simulink model "uz_interlockDeadtime2L"  (R2023a)
settings: Solver=FixedStepDiscrete  StartTime=0.0  StopTime=0.003  RelTol=1e-3
undefined symbols (not defined in the file or in its folder): f_FPGA_clk, T_FPGA_clk
libraries: simulink x3, hdlsllib x3
(part 1 of 2)
settings Model: DataTypeOverride=Off  Creator=ts  LastModifiedBy=ts
settings SolverCC: AlgebraicLoopSolver=TrustRegion
settings DataIOCC: LimitDataPoints=on  SaveOutput=off  SaveTime=off
settings OptimizationCC: BlockReduction=off  ConditionallyExecuteInputs=off  DefaultParameterBehavior=Inlined  LifeSpan=inf
settings DebuggingCC: AlgebraicLoopMsg=error  SingleTaskRateTransMsg=error  UnconnectedInputMsg=warning  UnconnectedOutputMsg=warning  UnconnectedLineMsg=warning  AllowSymbolicDim=off  StrictBusMsg=ErrorOnBusTreatedAsVector  SFUnexpectedBacktrackingDiag=warning  SFNoUnconditionalDefaultTransitionDiag=warning  SFExecutionAtInitializationDiag=none  ArithmeticOperatorsInVariantConditions=warning
settings HardwareCC: ProdBitPerPointer=32  ProdBitPerSizeT=32  ProdBitPerPtrDiffT=32  ProdLargestAtomicFloat=None  ProdIntDivRoundTo=Undefined  ProdEndianess=Unspecified  ProdWordSize=32  ProdHWDeviceType=ASIC/FPGA->ASIC/FPGA  ProdEqTarget=off
settings ModelReferenceCC: EnableRefExpFcnMdlSchedulingChecks=on
settings SFSimCC: SimUseLocalCustomCode=off  CustomCodeUndefinedFunction=UseInterfaceOnly
settings RTWCC: RTWUseLocalCustomCode=off  DLArmComputeVersion=19.05
settings CodeAppCC: StateflowObjectComments=on
settings GRTTargetCC: TargetLangStandard=C89/C90 (ANSI)
settings ConfigComp: CovScope=ReferencedModels  CovMetricSettings=dw  CovSaveCumulativeToWorkspaceVar=on  CovSaveSingleToWorkspaceVar=on  CovExternalEMLEnable=off  CovSFcnEnable=off

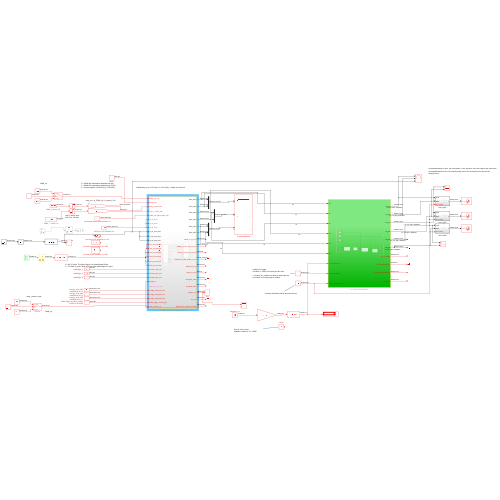
[thumbnail: Simulink's stored preview of the top-level diagram]
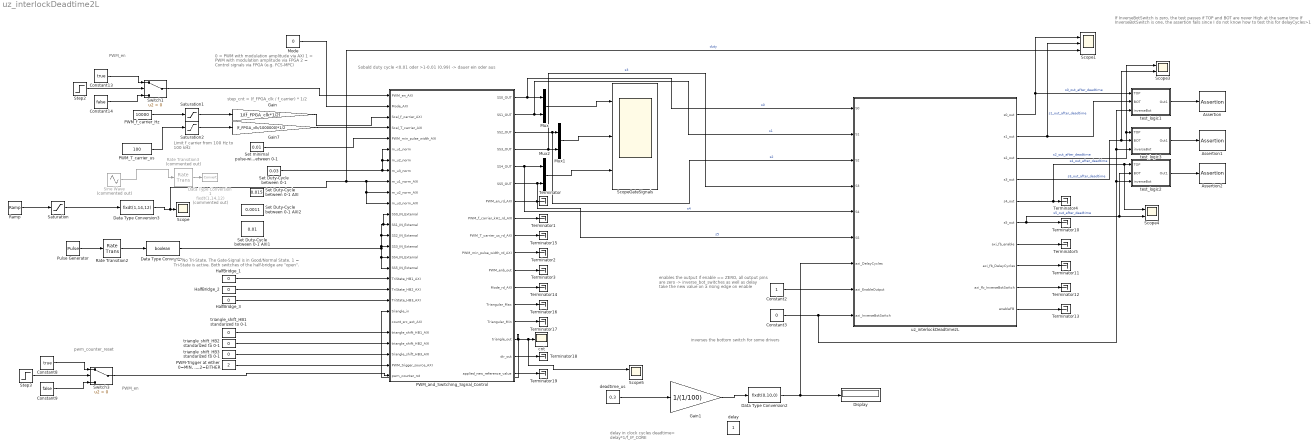
== system uz_interlockDeadtime2L ==
  note: Sobald duty cycle <0.01 oder >1-0.01 (0.99) -> dauer ein oder aus
  note: If InverseBotSwitch is zero, the test passes if TOP and BOT are never High at the same time
      | If InverseBotSwitch is one, the assertion fails since I do not know how to test this for delayCycles>1
  note: enables the output
      | if enable == ZERO, all output pins are zero
      |
      | -> inverse_bot_switches as well as delay take the
      | new value on a rising edge on enable
  note: inverses the bottom switch for some drivers
  note: delay in clock cycles
      | deadtime= delay*1/f_IP_CORE
  note: 0 = No Tri-State. The Gate-Signal is in Good/Normal State.
      | 1 = Tri-State is active. Both switches of the half-bridge are "open".
  note: 0 = PWM with modulation amplitude via AXI
      | 1 = PWM with modulation amplitude via FPGA
      | 2 = Control signals via FPGA (e.g. FCS-MPC)
  note: PWM_en
  note: Limit f_carrier from
      | 100 Hz to 100 kHz
  note: PWM_en
  note: step_cnt = (f_FPGA_clk / f_carrier) * 1/2
  note: pwm_counter_reset
  Assertion : Assertion
  Assertion1 : Assertion
  Assertion2 : Assertion
  Constant13 : Constant  Value=true  SampleTime=T_FPGA_clk
  Constant14 : Constant  Value=false  SampleTime=T_FPGA_clk
  Constant2 : Constant  OutDataTypeStr=boolean  SampleTime=1/100e6
  Constant3 : Constant  Value=0  OutDataTypeStr=boolean  SampleTime=1/100e6
  Constant8 : Constant  Value=true  SampleTime=T_FPGA_clk
  Constant9 : Constant  Value=false  SampleTime=T_FPGA_clk
  Data Type Conversion : DataTypeConversion  OutDataTypeStr=boolean  SaturateOnIntegerOverflow=off  RndMeth=Floor
  Data Type Conversion1 : DataTypeConversion  Commented=on  OutDataTypeStr=fixdt(1,14,12)  SaturateOnIntegerOverflow=off  RndMeth=Floor
  Data Type Conversion2 : DataTypeConversion  OutDataTypeStr=fixdt(0,10,0)  SaturateOnIntegerOverflow=off  RndMeth=Floor
  Data Type Conversion3 : DataTypeConversion  OutDataTypeStr=fixdt(1,14,12)  SaturateOnIntegerOverflow=off  RndMeth=Floor
  Display : Display
  Gain : Gain  Gain=1/(f_FPGA_clk*1/2)  OutDataTypeStr=fixdt(0,25,26)
  Gain1 : Gain  Gain=1/(1/100)
  Gain7 : Gain  Gain=(f_FPGA_clk/1000000)*1/2  OutDataTypeStr=fixdt(0,25,0)
  HalfBridge_1 : Constant  Value=0  OutDataTypeStr=fixdt(0,2,0)  SampleTime=T_FPGA_clk
  HalfBridge_2 : Constant  Value=0  OutDataTypeStr=fixdt(0,2,0)  SampleTime=T_FPGA_clk
  HalfBridge_3 : Constant  Value=0  OutDataTypeStr=fixdt(0,2,0)  SampleTime=T_FPGA_clk
  Mode : Constant  Value=0  OutDataTypeStr=fixdt(0,2,0)  SampleTime=T_FPGA_clk
  Mux : Mux  Inputs=2
  Mux1 : Mux  Inputs=2
  Mux2 : Mux  Inputs=2
  "PWM-Trigger at either 0=MIN, 1=MAX,2=EITHER" : Constant  Value=2  OutDataTypeStr=uint32  SampleTime=T_FPGA_clk
  PWM_T_carrier_us : Constant  Value=100  OutDataTypeStr=uint32  SampleTime=T_FPGA_clk
  PWM_and_Switching_Signal_Control : Subsystem  TreatAsAtomicUnit=on
  PWM_f_carrier_Hz : Constant  Value=10000  OutDataTypeStr=uint32  SampleTime=T_FPGA_clk
  Pulse Generator : DiscretePulseGenerator  PulseType=Time based  Period=0.01  PulseWidth=5
  Ramp : simulink/Sources/Ramp  slope=0.0000001/T_FPGA_clk  start=T_FPGA_clk  InitialOutput=0.97
  Rate Transition2 : RateTransition  OutPortSampleTime=T_FPGA_clk
  Rate Transition3 : RateTransition  Commented=on  OutPortSampleTime=T_FPGA_clk
  Saturation : Saturate  UpperLimit=1  LowerLimit=0
  Saturation1 : Saturate  UpperLimit=100000  LowerLimit=100
  Saturation2 : Saturate  UpperLimit=10000  LowerLimit=10
  Scope : Scope
  Scope1 : Scope  NumInputPorts=3
  Scope3 : Scope  NumInputPorts=2
  Scope4 : Scope  NumInputPorts=2
  Scope5 : Scope  NumInputPorts=2
  ScopeGateSignals : Scope  NumInputPorts=3
  Set Duty-Cycle between 0-1 : Constant  Value=0.03  OutDataTypeStr=fixdt(1,14,12)  SampleTime=T_FPGA_clk
  Set Duty-Cycle between 0-1 AXI : Constant  Value=0.015  OutDataTypeStr=fixdt(1,14,12)  SampleTime=T_FPGA_clk
  Set Duty-Cycle between 0-1 AXI1 : Constant  Value=0.01  OutDataTypeStr=fixdt(1,14,12)  SampleTime=T_FPGA_clk
  Set Duty-Cycle between 0-1 AXI2 : Constant  Value=0.0011  OutDataTypeStr=fixdt(1,14,12)  SampleTime=T_FPGA_clk
  Set minimal pulse-width between 0-1 : Constant  Value=0.01  OutDataTypeStr=fixdt(1,18,16)  SampleTime=T_FPGA_clk
  Sine Wave : Sin  Commented=on  Frequency=500  SampleTime=0
  Step2 : Step  Time=0.002  Before=1  SampleTime=T_FPGA_clk
  Step3 : Step  Time=0.00025  After=0  SampleTime=T_FPGA_clk
  Switch1 : Switch  Criteria=u2 > Threshold  SaturateOnIntegerOverflow=off  InputSameDT=off
  Switch3 : Switch  Criteria=u2 > Threshold  SaturateOnIntegerOverflow=off  InputSameDT=off
  Terminator{,1..5,10..19} (16 alike) : Terminator
  cnt : Scope
  deadtime_us : Constant  Value=0.3  OutDataTypeStr=double  SampleTime=1/100e6
  delay : Constant  OutDataTypeStr=fixdt(0,10,0)  SampleTime=1/100e6
  test_logic1 : Subsystem
  test_logic2 : Subsystem
  test_logic3 : Subsystem
  triangle_shift_HB1 standarized to 0-1 : Constant  Value=0  OutDataTypeStr=fixdt(0,18,17)  SampleTime=T_FPGA_clk
  triangle_shift_HB2 standarized to 0-1 : Constant  Value=0  OutDataTypeStr=fixdt(0,18,17)  SampleTime=T_FPGA_clk
  triangle_shift_HB3 standarized to 0-1 : Constant  Value=0  OutDataTypeStr=fixdt(0,18,17)  SampleTime=T_FPGA_clk
  uz_interlockDeadtime2L : Subsystem  TreatAsAtomicUnit=on
  wires:
  Constant2/1 -> uz_interlockDeadtime2L/8(axi_EnableOutput)
  uz_interlockDeadtime2L/1(s0_out) -> Scope1/1, test_logic1/1(TOP)  "s0_out_after_deadtime"
  uz_interlockDeadtime2L/2(s1_out) -> Scope1/2, test_logic1/2(BOT)  "s1_out_after_deadtime"
  uz_interlockDeadtime2L/3(s2_out) -> Scope3/1, test_logic3/1(TOP)  "s2_out_after_deadtime"
  uz_interlockDeadtime2L/4(s3_out) -> Scope3/2, test_logic3/2(BOT)  "s3_out_after_deadtime"
  uz_interlockDeadtime2L/5(s4_out) -> Scope4/1, test_logic2/1(TOP), Terminator4/1  "s4_out_after_deadtime"
  Constant3/1 -> uz_interlockDeadtime2L/9(axi_InverseBotSwitch), test_logic2/3(inverseBot), test_logic3/3(inverseBot), test_logic1/3(inverseBot)
  uz_interlockDeadtime2L/6(s5_out) -> test_logic2/2(BOT), Scope4/2, Terminator10/1  "s5_out_after_deadtime"
  uz_interlockDeadtime2L/7(axi_fb_enable) -> Terminator5/1
  uz_interlockDeadtime2L/8(axi_fb_DelayCycles) -> Terminator11/1
  uz_interlockDeadtime2L/9(axi_fb_InverseBotSwitch) -> Terminator12/1
  uz_interlockDeadtime2L/10(enableFB) -> Terminator13/1
  test_logic3/1(Out1) -> Assertion1/1
  test_logic2/1(Out1) -> Assertion2/1
  test_logic1/1(Out1) -> Assertion/1
  Data Type Conversion2/1 -> Display/1, uz_interlockDeadtime2L/7(axi_DelayCycles)
  PWM_and_Switching_Signal_Control/13(Triangular_Max) -> Terminator16/1
  triangle_shift_HB3 standarized to 0-1/1 -> PWM_and_Switching_Signal_Control/25(triangle_shift_HB3_AXI)
  PWM_and_Switching_Signal_Control/8(PWM_f_carrier_kHz_rd_AXI) -> Terminator1/1
  triangle_shift_HB1 standarized to 0-1/1 -> PWM_and_Switching_Signal_Control/23(triangle_shift_HB1_AXI)
  PWM_and_Switching_Signal_Control/7(PWM_en_rd_AXI) -> Terminator/1
  PWM_and_Switching_Signal_Control/15(triangle_out) -> PWM_and_Switching_Signal_Control/21(triangle_in), Scope5/1, cnt/1
  PWM_and_Switching_Signal_Control/2(SS1_OUT) -> uz_interlockDeadtime2L/2(S1), Mux/2  "s1"
  Constant9/1 -> Switch3/3
  Constant14/1 -> Switch1/3
  "PWM-Trigger at either 0=MIN, 1=MAX,2=EITHER"/1 -> PWM_and_Switching_Signal_Control/26(PWM_trigger_source_AXI)
  Switch1/1 -> PWM_and_Switching_Signal_Control/1(PWM_en_AXI)
  Set Duty-Cycle between 0-1/1 -> PWM_and_Switching_Signal_Control/6(m_u1_norm), PWM_and_Switching_Signal_Control/7(m_u2_norm), PWM_and_Switching_Signal_Control/8(m_u3_norm)
  Mux/1 -> ScopeGateSignals/1
  Data Type Conversion/1 -> PWM_and_Switching_Signal_Control/13(SS1_IN_External), PWM_and_Switching_Signal_Control/12(SS0_IN_External), PWM_and_Switching_Signal_Control/14(SS2_IN_External), PWM_and_Switching_Signal_Control/15(SS3_IN_External), PWM_and_Switching_Signal_Control/17(SS5_IN_External), PWM_and_Switching_Signal_Control/16(SS4_IN_External)
  Mode/1 -> PWM_and_Switching_Signal_Control/2(Mode_AXI)
  Gain/1 -> PWM_and_Switching_Signal_Control/3(Scal_f_carrier_AXI)
  Pulse Generator/1 -> Rate Transition2/1
  Constant8/1 -> Switch3/1
  PWM_and_Switching_Signal_Control/14(Triangular_Min) -> Terminator17/1
  HalfBridge_3/1 -> PWM_and_Switching_Signal_Control/20(TriState_HB3_AXI)
  Mux2/1 -> ScopeGateSignals/3
  PWM_T_carrier_us/1 -> Saturation2/1
  Saturation2/1 -> Gain7/1
  PWM_and_Switching_Signal_Control/11(PWM_enb_out) -> Terminator3/1
  PWM_and_Switching_Signal_Control/9(PWM_T_carrier_us_rd_AXI) -> Terminator15/1
  Rate Transition3/1 -> Data Type Conversion1/1
  PWM_and_Switching_Signal_Control/12(Mode_rd_AXI) -> Terminator14/1
  PWM_and_Switching_Signal_Control/16(dir_out) -> Terminator18/1
  Rate Transition2/1 -> Data Type Conversion/1
  HalfBridge_1/1 -> PWM_and_Switching_Signal_Control/18(TriState_HB1_AXI)
  PWM_and_Switching_Signal_Control/17(applied_new_reference_value) -> Terminator19/1
  PWM_and_Switching_Signal_Control/4(SS3_OUT) -> uz_interlockDeadtime2L/4(S3), Mux1/2  "s3"
  Mux1/1 -> ScopeGateSignals/2
  PWM_and_Switching_Signal_Control/6(SS5_OUT) -> uz_interlockDeadtime2L/6(S5), Mux2/2  "s5"
  PWM_and_Switching_Signal_Control/10(PWM_min_pulse_width_rd_AXI) -> Terminator2/1
  HalfBridge_2/1 -> PWM_and_Switching_Signal_Control/19(TriState_HB2_AXI)
  Constant13/1 -> Switch1/1
  PWM_and_Switching_Signal_Control/5(SS4_OUT) -> uz_interlockDeadtime2L/5(S4), Mux2/1  "s4"
  Gain7/1 -> PWM_and_Switching_Signal_Control/4(Scal_T_carrier_AXI)
  Step3/1 -> Switch3/2
  Sine Wave/1 -> Rate Transition3/1
  Switch3/1 -> PWM_and_Switching_Signal_Control/27(pwm_counter_rst)
  PWM_and_Switching_Signal_Control/1(SS0_OUT) -> uz_interlockDeadtime2L/1(S0), Mux/1  "s0"
  Data Type Conversion3/1 -> Scope1/3, PWM_and_Switching_Signal_Control/11(m_u3_norm_AXI), PWM_and_Switching_Signal_Control/10(m_u2_norm_AXI), PWM_and_Switching_Signal_Control/9(m_u1_norm_AXI), Scope/1  "duty"
  PWM_and_Switching_Signal_Control/3(SS2_OUT) -> uz_interlockDeadtime2L/3(S2), Mux1/1  "s2"
  triangle_shift_HB2 standarized to 0-1/1 -> PWM_and_Switching_Signal_Control/24(triangle_shift_HB2_AXI)
  Saturation1/1 -> Gain/1
  Step2/1 -> Switch1/2
  PWM_f_carrier_Hz/1 -> Saturation1/1
  Set minimal pulse-width between 0-1/1 -> PWM_and_Switching_Signal_Control/5(PWM_min_pulse_width_AXI)
  deadtime_us/1 -> Gain1/1
  Gain1/1 -> Data Type Conversion2/1
  Ramp/1 -> Saturation/1
  Saturation/1 -> Data Type Conversion3/1

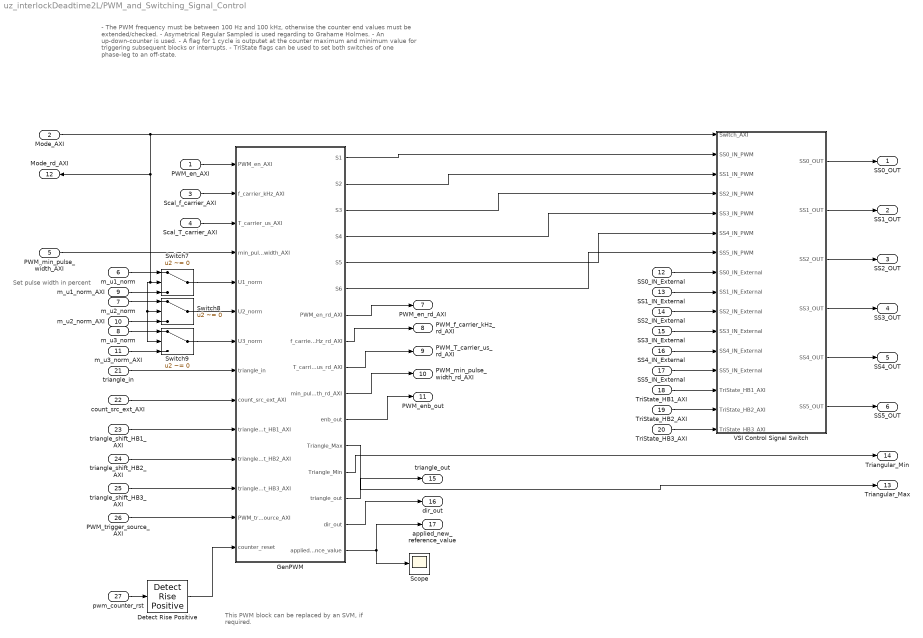
== system uz_interlockDeadtime2L/PWM_and_Switching_Signal_Control ==
  note: This PWM block can be replaced by an SVM,
      | if required.
  note: - The PWM frequency must be between 100 Hz and 100 kHz, otherwise the counter end values must be extended/checked.
      | - Asymetrical Regular Sampled is used regarding to Grahame Holmes.
      | - An up-down-counter is used.
      | - A flag for 1 cycle is outputet at the counter maximum and minimum value for triggering subsequent blocks or interrupts.
      | - TriState flags can be used to set both switches of one phase-leg to an off-state.
  note: Set pulse width in percent
  PWM_en_AXI : Inport
  Mode_AXI : Inport  Port=2
  Scal_f_carrier_AXI : Inport  Port=3
  Scal_T_carrier_AXI : Inport  Port=4
  PWM_min_pulse_width_AXI : Inport  Port=5
  m_u1_norm : Inport  Port=6
  m_u2_norm : Inport  Port=7
  m_u3_norm : Inport  Port=8
  m_u1_norm_AXI : Inport  Port=9
  m_u2_norm_AXI : Inport  Port=10
  m_u3_norm_AXI : Inport  Port=11
  SS0_IN_External : Inport  Port=12
  SS1_IN_External : Inport  Port=13
  SS2_IN_External : Inport  Port=14
  SS3_IN_External : Inport  Port=15
  SS4_IN_External : Inport  Port=16
  SS5_IN_External : Inport  Port=17
  TriState_HB1_AXI : Inport  Port=18
  TriState_HB2_AXI : Inport  Port=19
  TriState_HB3_AXI : Inport  Port=20
  triangle_in : Inport  Port=21
  count_src_ext_AXI : Inport  Port=22
  triangle_shift_HB1_AXI : Inport  Port=23
  triangle_shift_HB2_AXI : Inport  Port=24
  triangle_shift_HB3_AXI : Inport  Port=25
  PWM_trigger_source_AXI : Inport  Port=26
  pwm_counter_rst : Inport  Port=27
  Detect Rise Positive : simulink/Logic and Bit Operations/Detect Rise Positive  vinit=0  OutDataTypeStr=boolean
  GenPWM : Subsystem  TreatAsAtomicUnit=on
  Scope : Scope
  Switch7 : Switch  Criteria=u2 ~= 0  SaturateOnIntegerOverflow=off  InputSameDT=off
  Switch8 : Switch  Criteria=u2 ~= 0  SaturateOnIntegerOverflow=off  InputSameDT=off
  Switch9 : Switch  Criteria=u2 ~= 0  SaturateOnIntegerOverflow=off  InputSameDT=off
  VSI Control Signal Switch : Subsystem
  SS0_OUT : Outport  VectorParamsAs1DForOutWhenUnconnected=off
  SS1_OUT : Outport  Port=2  VectorParamsAs1DForOutWhenUnconnected=off
  SS2_OUT : Outport  Port=3  VectorParamsAs1DForOutWhenUnconnected=off
  SS3_OUT : Outport  Port=4  VectorParamsAs1DForOutWhenUnconnected=off
  SS4_OUT : Outport  Port=5  VectorParamsAs1DForOutWhenUnconnected=off
  SS5_OUT : Outport  Port=6  VectorParamsAs1DForOutWhenUnconnected=off
  PWM_en_rd_AXI : Outport  Port=7  VectorParamsAs1DForOutWhenUnconnected=off
  PWM_f_carrier_kHz_rd_AXI : Outport  Port=8  VectorParamsAs1DForOutWhenUnconnected=off
  PWM_T_carrier_us_rd_AXI : Outport  Port=9  VectorParamsAs1DForOutWhenUnconnected=off
  PWM_min_pulse_width_rd_AXI : Outport  Port=10  VectorParamsAs1DForOutWhenUnconnected=off
  PWM_enb_out : Outport  Port=11  VectorParamsAs1DForOutWhenUnconnected=off
  Mode_rd_AXI : Outport  Port=12  VectorParamsAs1DForOutWhenUnconnected=off
  Triangular_Max : Outport  Port=13  VectorParamsAs1DForOutWhenUnconnected=off
  Triangular_Min : Outport  Port=14  VectorParamsAs1DForOutWhenUnconnected=off
  triangle_out : Outport  Port=15  VectorParamsAs1DForOutWhenUnconnected=off
  dir_out : Outport  Port=16  VectorParamsAs1DForOutWhenUnconnected=off
  applied_new_reference_value : Outport  Port=17  VectorParamsAs1DForOutWhenUnconnected=off
  wires:
  VSI Control Signal Switch/1(SS0_OUT) -> SS0_OUT/1
  Mode_AXI/1 -> Mode_rd_AXI/1, Switch9/2, Switch8/2, Switch7/2, VSI Control Signal Switch/1(Switch_AXI)
  GenPWM/4(S4) -> VSI Control Signal Switch/5(SS3_IN_PWM)
  Scal_f_carrier_AXI/1 -> GenPWM/2(f_carrier_kHz_AXI)
  GenPWM/2(S2) -> VSI Control Signal Switch/3(SS1_IN_PWM)
  SS1_IN_External/1 -> VSI Control Signal Switch/9(SS1_IN_External)
  GenPWM/3(S3) -> VSI Control Signal Switch/4(SS2_IN_PWM)
  GenPWM/5(S5) -> VSI Control Signal Switch/6(SS4_IN_PWM)
  GenPWM/6(S6) -> VSI Control Signal Switch/7(SS5_IN_PWM)
  VSI Control Signal Switch/6(SS5_OUT) -> SS5_OUT/1
  GenPWM/1(S1) -> VSI Control Signal Switch/2(SS0_IN_PWM)
  GenPWM/11(enb_out) -> PWM_enb_out/1
  VSI Control Signal Switch/3(SS2_OUT) -> SS2_OUT/1
  SS3_IN_External/1 -> VSI Control Signal Switch/11(SS3_IN_External)
  SS0_IN_External/1 -> VSI Control Signal Switch/8(SS0_IN_External)
  VSI Control Signal Switch/2(SS1_OUT) -> SS1_OUT/1
  SS4_IN_External/1 -> VSI Control Signal Switch/12(SS4_IN_External)
  PWM_en_AXI/1 -> GenPWM/1(PWM_en_AXI)
  SS5_IN_External/1 -> VSI Control Signal Switch/13(SS5_IN_External)
  VSI Control Signal Switch/5(SS4_OUT) -> SS4_OUT/1
  PWM_min_pulse_width_AXI/1 -> GenPWM/4(min_pulse_width_AXI)
  SS2_IN_External/1 -> VSI Control Signal Switch/10(SS2_IN_External)
  VSI Control Signal Switch/4(SS3_OUT) -> SS3_OUT/1
  Switch9/1 -> GenPWM/7(U3_norm)
  m_u1_norm_AXI/1 -> Switch7/3
  m_u1_norm/1 -> Switch7/1
  m_u2_norm/1 -> Switch8/1
  m_u2_norm_AXI/1 -> Switch8/3
  m_u3_norm/1 -> Switch9/1
  m_u3_norm_AXI/1 -> Switch9/3
  GenPWM/7(PWM_en_rd_AXI) -> PWM_en_rd_AXI/1
  GenPWM/8(f_carrier_kHz_rd_AXI) -> PWM_f_carrier_kHz_rd_AXI/1
  GenPWM/10(min_pulse_width_rd_AXI) -> PWM_min_pulse_width_rd_AXI/1
  GenPWM/9(T_carrier_us_rd_AXI) -> PWM_T_carrier_us_rd_AXI/1
  Switch8/1 -> GenPWM/6(U2_norm)
  Switch7/1 -> GenPWM/5(U1_norm)
  Scal_T_carrier_AXI/1 -> GenPWM/3(T_carrier_us_AXI)
  GenPWM/12(Triangle_Max) -> Triangular_Max/1
  TriState_HB1_AXI/1 -> VSI Control Signal Switch/14(TriState_HB1_AXI)
  TriState_HB2_AXI/1 -> VSI Control Signal Switch/15(TriState_HB2_AXI)
  TriState_HB3_AXI/1 -> VSI Control Signal Switch/16(TriState_HB3_AXI)
  GenPWM/13(Triangle_Min) -> Triangular_Min/1
  triangle_in/1 -> GenPWM/8(triangle_in)
  GenPWM/14(triangle_out) -> triangle_out/1
  GenPWM/15(dir_out) -> dir_out/1
  count_src_ext_AXI/1 -> GenPWM/9(count_src_ext_AXI)
  triangle_shift_HB1_AXI/1 -> GenPWM/10(triangle_shift_HB1_AXI)
  triangle_shift_HB3_AXI/1 -> GenPWM/12(triangle_shift_HB3_AXI)
  triangle_shift_HB2_AXI/1 -> GenPWM/11(triangle_shift_HB2_AXI)
  PWM_trigger_source_AXI/1 -> GenPWM/13(PWM_trigger_source_AXI)
  GenPWM/16(applied_new_reference_value) -> Scope/1, applied_new_reference_value/1
  Detect Rise Positive/1 -> GenPWM/14(counter_reset)
  pwm_counter_rst/1 -> Detect Rise Positive/1

== system uz_interlockDeadtime2L/test_logic1 ==
  TOP : Inport
  BOT : Inport  Port=2
  inverseBot : Inport  Port=3
  AND : Logic  IconShape=distinctive  AllPortsSameDT=off  OutDataTypeStr=boolean
  Constant : Constant
  NOT : Logic  Operator=NOT  IconShape=distinctive  AllPortsSameDT=off  OutDataTypeStr=boolean
  Switch : Switch  Criteria=u2 ~= 0  SaturateOnIntegerOverflow=off  InputSameDT=off
  Out1 : Outport
  wires:
  Constant/1 -> Switch/1
  Switch/1 -> Out1/1
  AND/1 -> NOT/1
  inverseBot/1 -> Switch/2
  NOT/1 -> Switch/3
  TOP/1 -> AND/1
  BOT/1 -> AND/2

== system uz_interlockDeadtime2L/test_logic2 ==
  TOP : Inport
  BOT : Inport  Port=2
  inverseBot : Inport  Port=3
  AND : Logic  IconShape=distinctive  AllPortsSameDT=off  OutDataTypeStr=boolean
  Constant : Constant
  NOT : Logic  Operator=NOT  IconShape=distinctive  AllPortsSameDT=off  OutDataTypeStr=boolean
  Switch : Switch  Criteria=u2 ~= 0  SaturateOnIntegerOverflow=off  InputSameDT=off
  Out1 : Outport
  wires:
  BOT/1 -> AND/2
  TOP/1 -> AND/1
  NOT/1 -> Switch/3
  inverseBot/1 -> Switch/2
  AND/1 -> NOT/1
  Switch/1 -> Out1/1
  Constant/1 -> Switch/1

== system uz_interlockDeadtime2L/test_logic3 ==
  TOP : Inport
  BOT : Inport  Port=2
  inverseBot : Inport  Port=3
  AND : Logic  IconShape=distinctive  AllPortsSameDT=off  OutDataTypeStr=boolean
  Constant : Constant
  NOT : Logic  Operator=NOT  IconShape=distinctive  AllPortsSameDT=off  OutDataTypeStr=boolean
  Switch : Switch  Criteria=u2 ~= 0  SaturateOnIntegerOverflow=off  InputSameDT=off
  Out1 : Outport
  wires:
  Constant/1 -> Switch/1
  Switch/1 -> Out1/1
  AND/1 -> NOT/1
  inverseBot/1 -> Switch/2
  NOT/1 -> Switch/3
  TOP/1 -> AND/1
  BOT/1 -> AND/2

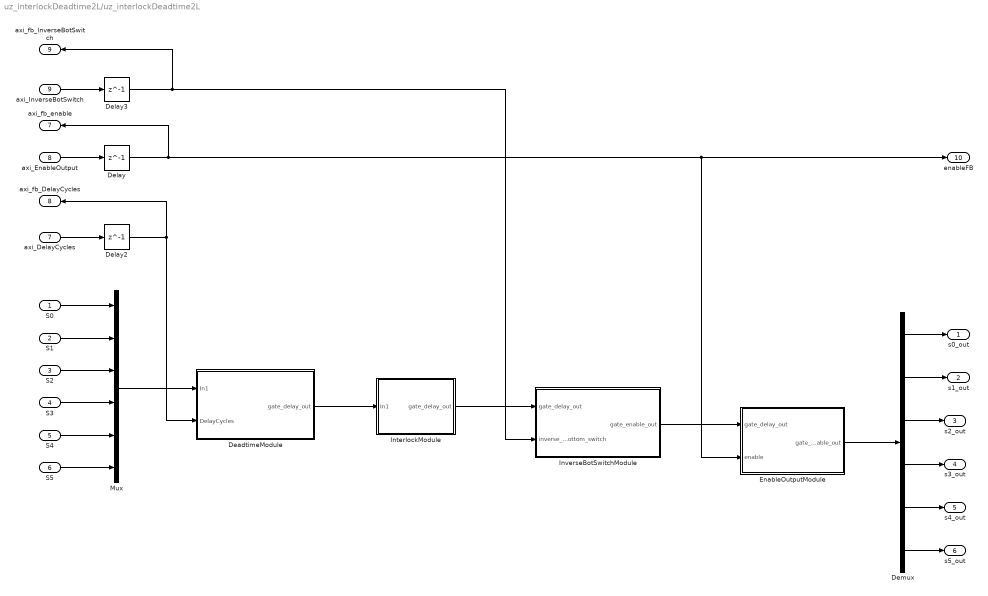
== system uz_interlockDeadtime2L/uz_interlockDeadtime2L ==
  S0 : Inport
  S1 : Inport  Port=2
  S2 : Inport  Port=3
  S3 : Inport  Port=4
  S4 : Inport  Port=5
  S5 : Inport  Port=6
  axi_DelayCycles : Inport  Port=7
  axi_EnableOutput : Inport  Port=8
  axi_InverseBotSwitch : Inport  Port=9
  DeadtimeModule : Subsystem  TreatAsAtomicUnit=on
  Delay : Delay  DelayLength=1
  Delay2 : Delay  DelayLength=1
  Delay3 : Delay  DelayLength=1
  Demux : Demux  Outputs=6
  EnableOutputModule : Subsystem  TreatAsAtomicUnit=on
  InterlockModule : Subsystem  TreatAsAtomicUnit=on
  InverseBotSwitchModule : Subsystem  TreatAsAtomicUnit=on
  Mux : Mux  Inputs=6
  s0_out : Outport  VectorParamsAs1DForOutWhenUnconnected=off
  s1_out : Outport  Port=2  VectorParamsAs1DForOutWhenUnconnected=off
  s2_out : Outport  Port=3  VectorParamsAs1DForOutWhenUnconnected=off
  s3_out : Outport  Port=4  VectorParamsAs1DForOutWhenUnconnected=off
  s4_out : Outport  Port=5  VectorParamsAs1DForOutWhenUnconnected=off
  s5_out : Outport  Port=6  VectorParamsAs1DForOutWhenUnconnected=off
  axi_fb_enable : Outport  Port=7  VectorParamsAs1DForOutWhenUnconnected=off
  axi_fb_DelayCycles : Outport  Port=8  VectorParamsAs1DForOutWhenUnconnected=off
  axi_fb_InverseBotSwitch : Outport  Port=9  VectorParamsAs1DForOutWhenUnconnected=off
  enableFB : Outport  Port=10  VectorParamsAs1DForOutWhenUnconnected=off
  wires:
  axi_InverseBotSwitch/1 -> Delay3/1
  Delay3/1 -> InverseBotSwitchModule/2(inverse_bottom_switch), axi_fb_InverseBotSwitch/1
  axi_EnableOutput/1 -> Delay/1
  Delay2/1 -> axi_fb_DelayCycles/1, DeadtimeModule/2(DelayCycles)
  Mux/1 -> DeadtimeModule/1(In1)
  DeadtimeModule/1(gate_delay_out) -> InterlockModule/1(In1)
  S0/1 -> Mux/1
  S1/1 -> Mux/2
  S2/1 -> Mux/3
  S3/1 -> Mux/4
  S4/1 -> Mux/5
  S5/1 -> Mux/6
  Demux/2 -> s1_out/1
  Demux/1 -> s0_out/1
  Demux/3 -> s2_out/1
  Demux/4 -> s3_out/1
  Demux/5 -> s4_out/1
  Demux/6 -> s5_out/1
  EnableOutputModule/1(gate_enable_out) -> Demux/1
  Delay/1 -> axi_fb_enable/1, enableFB/1, EnableOutputModule/2(enable)
  InterlockModule/1(gate_delay_out) -> InverseBotSwitchModule/1(gate_delay_out)
  InverseBotSwitchModule/1(gate_enable_out) -> EnableOutputModule/1(gate_delay_out)
  axi_DelayCycles/1 -> Delay2/1

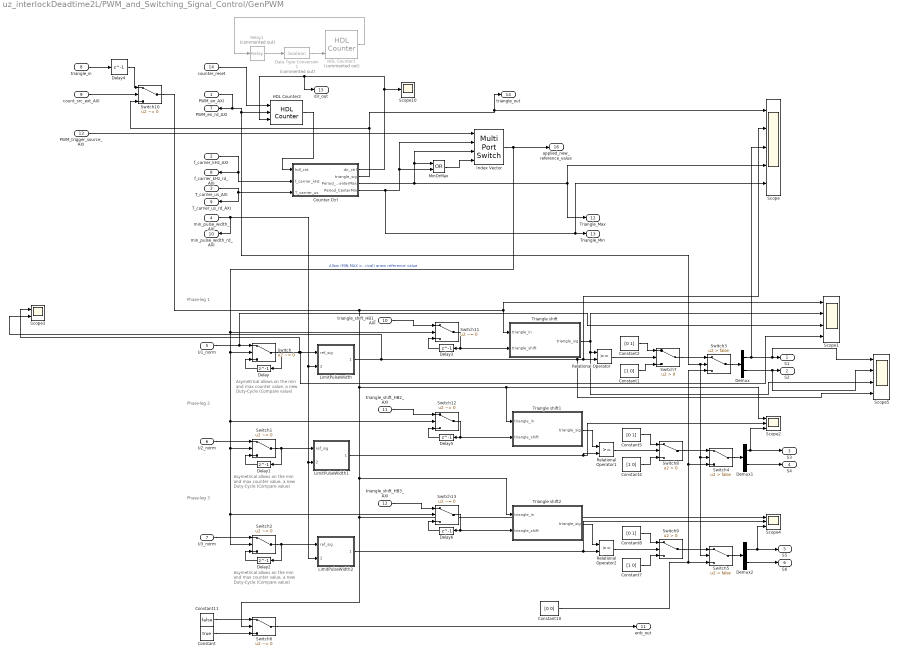
== system uz_interlockDeadtime2L/PWM_and_Switching_Signal_Control/GenPWM ==
  note: Asymetrical allows on the min
      |  and max counter value, a new
      |  Duty-Cycle (Compare value)
  note: Phase-leg 1
  note: Phase-leg 2
  note: Phase-leg 3
  note: Asymetrical allows on the min
      |  and max counter value, a new
      |  Duty-Cycle (Compare value)
  note: Asymetrical allows on the min
      |  and max counter value, a new
      |  Duty-Cycle (Compare value)
  PWM_en_AXI : Inport
  f_carrier_kHz_AXI : Inport  Port=2
  T_carrier_us_AXI : Inport  Port=3
  min_pulse_width_AXI : Inport  Port=4
  U1_norm : Inport  Port=5
  U2_norm : Inport  Port=6
  U3_norm : Inport  Port=7
  triangle_in : Inport  Port=8
  count_src_ext_AXI : Inport  Port=9
  triangle_shift_HB1_AXI : Inport  Port=10
  triangle_shift_HB2_AXI : Inport  Port=11
  triangle_shift_HB3_AXI : Inport  Port=12
  PWM_trigger_source_AXI : Inport  Port=13
  counter_reset : Inport  Port=14
  Constant : Constant  Value=true  SampleTime=T_FPGA_clk
  Constant1 : Constant  Value=[1 0]  OutDataTypeStr=fixdt(0,1,0)  SampleTime=T_FPGA_clk
  Constant10 : Constant  Value=[0 0]  OutDataTypeStr=fixdt(0,1,0)  SampleTime=T_FPGA_clk
  Constant11 : Constant  Value=false  SampleTime=T_FPGA_clk
  Constant2 : Constant  Value=[0 1]  OutDataTypeStr=fixdt(0,1,0)  SampleTime=T_FPGA_clk
  Constant4 : Constant  Value=[1 0]  OutDataTypeStr=fixdt(0,1,0)  SampleTime=T_FPGA_clk
  Constant5 : Constant  Value=[0 1]  OutDataTypeStr=fixdt(0,1,0)  SampleTime=T_FPGA_clk
  Constant7 : Constant  Value=[1 0]  OutDataTypeStr=fixdt(0,1,0)  SampleTime=T_FPGA_clk
  Constant8 : Constant  Value=[0 1]  OutDataTypeStr=fixdt(0,1,0)  SampleTime=T_FPGA_clk
  Counter Ctrl : Subsystem
  Data Type Conversion1 : DataTypeConversion  Commented=on  OutDataTypeStr=boolean  SaturateOnIntegerOverflow=off  RndMeth=Floor
  Delay{,1..6} (7 alike) : Delay  DelayLength=1
  Demux : Demux  Outputs=2
  Demux1 : Demux  Outputs=2
  Demux2 : Demux  Outputs=2
  HDL Counter1 : hdlsllib/Sources/HDL Counter  Commented=on  CountType=Free running  CountInit=0  CountStep=1  CountMax=100  CountFromType=Initial value  CountFrom=0  CountResetPort=on  CountLoadPort=off  CountEnbPort=on  CountDirPort=on  CountHitOutputPort=off  CountDataType=Signed  CountWordLen=8  CountFracLen=0  CountSampTime=Ts
  HDL Counter2 : hdlsllib/Sources/HDL Counter  CountType=Free running  CountInit=0  CountStep=1  CountMax=100  CountFromType=Initial value  CountFrom=0  CountResetPort=on  CountLoadPort=off  CountEnbPort=on  CountDirPort=on  CountHitOutputPort=off  CountDataType=Unsigned  CountWordLen=20  CountFracLen=0  CountSampTime=1
  Index Vector : MultiPortSwitch  DataPortOrder=Zero-based contiguous  zeroidx=on  SaturateOnIntegerOverflow=off  InputSameDT=off
  LimitPulseWidth : Subsystem
  LimitPulseWidth1 : Subsystem
  LimitPulseWidth2 : Subsystem
  MinOrMax : Logic  Operator=OR  AllPortsSameDT=off  OutDataTypeStr=boolean
  Relational Operator : RelationalOperator  OutDataTypeStr=boolean  InputSameDT=off
  Relational Operator1 : RelationalOperator  OutDataTypeStr=boolean  InputSameDT=off
  Relational Operator2 : RelationalOperator  OutDataTypeStr=boolean  InputSameDT=off
  Relay1 : Relay  Commented=on  OnSwitchValue=100  OffSwitchValue=0  OnOutputValue=0  OffOutputValue=1
  Scope : Scope  NumInputPorts=5
  Scope1 : Scope  NumInputPorts=4
  Scope10 : Scope
  Scope2 : Scope  NumInputPorts=3
  Scope3 : Scope  NumInputPorts=2
  Scope4 : Scope  NumInputPorts=3
  Scope5 : Scope  NumInputPorts=4
  Switch{,10..13} (5 alike) : Switch  Criteria=u2 ~= 0  Threshold=1  SaturateOnIntegerOverflow=off  InputSameDT=off
  Switch1 : Switch  Criteria=u2 ~= 0  SaturateOnIntegerOverflow=off  InputSameDT=off
  Switch2 : Switch  Criteria=u2 ~= 0  SaturateOnIntegerOverflow=off  InputSameDT=off
  Switch3 : Switch  Criteria=u2 > Threshold  Threshold=false  SaturateOnIntegerOverflow=off  InputSameDT=off
  Switch4 : Switch  Criteria=u2 > Threshold  Threshold=false  SaturateOnIntegerOverflow=off  InputSameDT=off
  Switch5 : Switch  Criteria=u2 > Threshold  Threshold=false  SaturateOnIntegerOverflow=off  InputSameDT=off
  Switch6 : Switch  Criteria=u2 ~= 0  SaturateOnIntegerOverflow=off  InputSameDT=off
  Switch7 : Switch  Criteria=u2 > Threshold  SaturateOnIntegerOverflow=off  InputSameDT=off
  Switch8 : Switch  Criteria=u2 > Threshold  SaturateOnIntegerOverflow=off  InputSameDT=off
  Switch9 : Switch  Criteria=u2 > Threshold  SaturateOnIntegerOverflow=off  InputSameDT=off
  Triangle shift : Subsystem
  Triangle shift1 : Subsystem
  Triangle shift2 : Subsystem
  S1 : Outport  VectorParamsAs1DForOutWhenUnconnected=off
  S2 : Outport  Port=2  VectorParamsAs1DForOutWhenUnconnected=off
  S3 : Outport  Port=3  VectorParamsAs1DForOutWhenUnconnected=off
  S4 : Outport  Port=4  VectorParamsAs1DForOutWhenUnconnected=off
  S5 : Outport  Port=5  VectorParamsAs1DForOutWhenUnconnected=off
  S6 : Outport  Port=6  VectorParamsAs1DForOutWhenUnconnected=off
  PWM_en_rd_AXI : Outport  Port=7  VectorParamsAs1DForOutWhenUnconnected=off
  f_carrier_kHz_rd_AXI : Outport  Port=8  VectorParamsAs1DForOutWhenUnconnected=off
  T_carrier_us_rd_AXI : Outport  Port=9  VectorParamsAs1DForOutWhenUnconnected=off
  min_pulse_width_rd_AXI : Outport  Port=10  VectorParamsAs1DForOutWhenUnconnected=off
  enb_out : Outport  Port=11  VectorParamsAs1DForOutWhenUnconnected=off
  Triangle_Max : Outport  Port=12  VectorParamsAs1DForOutWhenUnconnected=off
  Triangle_Min : Outport  Port=13  VectorParamsAs1DForOutWhenUnconnected=off
  triangle_out : Outport  Port=14  VectorParamsAs1DForOutWhenUnconnected=off
  dir_out : Outport  Port=15  VectorParamsAs1DForOutWhenUnconnected=off
  applied_new_reference_value : Outport  Port=16  OutDataTypeStr=boolean  VectorParamsAs1DForOutWhenUnconnected=off
  wires:
  Constant7/1 -> Switch9/3
  Demux2/2 -> S6/1
  Constant8/1 -> Switch9/1
  Relational Operator2/1 -> Switch9/2
  Switch9/1 -> Switch5/1
  Demux/2 -> Scope5/2, S2/1
  Relational Operator/1 -> Switch7/2
  Demux1/2 -> S4/1
  Constant5/1 -> Switch8/1
  Relational Operator1/1 -> Switch8/2
  Constant4/1 -> Switch8/3
  Constant1/1 -> Switch7/3
  Constant2/1 -> Switch7/1
  LimitPulseWidth/1(ref_sig_limit) -> Scope3/2, Scope5/4, Scope/2, Relational Operator/2
  LimitPulseWidth1/1(ref_sig_limit) -> Scope2/2, Relational Operator1/2
  LimitPulseWidth2/1(ref_sig_limit) -> Scope4/2, Relational Operator2/2
  Counter Ctrl/2(triangle_sig) -> triangle_out/1, Scope/1, Switch10/3
  PWM_en_AXI/1 -> Switch3/2, Switch4/2, Switch5/2, HDL Counter2/2, PWM_en_rd_AXI/1
  Delay/1 -> Switch/3
  Delay1/1 -> Switch1/3
  Delay2/1 -> Switch2/3
  Switch5/1 -> Demux2/1
  Switch8/1 -> Switch4/1
  Switch4/1 -> Demux1/1
  Switch3/1 -> Demux/1
  Constant10/1 -> Switch5/3, Switch3/3, Switch4/3
  U1_norm/1 -> Scope1/3, Switch/1
  U3_norm/1 -> Switch2/1
  U2_norm/1 -> Switch1/1
  Counter Ctrl/1(dir_ctrl) -> dir_out/1, HDL Counter2/3, Scope10/1
  f_carrier_kHz_AXI/1 -> f_carrier_kHz_rd_AXI/1, Counter Ctrl/2(f_carrier_kHz)
  Relay1/1 -> Data Type Conversion1/1
  Data Type Conversion1/1 -> HDL Counter1/3
  HDL Counter1/1 -> Relay1/1
  Switch/1 -> Delay/1, Scope3/1, Scope1/4, LimitPulseWidth/1(ref_sig)
  Switch1/1 -> LimitPulseWidth1/1(ref_sig), Delay1/1
  Switch2/1 -> LimitPulseWidth2/1(ref_sig), Delay2/1
  Demux/1 -> Scope/3, Scope5/1, S1/1
  Switch6/1 -> enb_out/1
  Constant11/1 -> Switch6/1
  Constant/1 -> Switch6/3
  Demux1/1 -> Scope2/3, S3/1
  Demux2/1 -> Scope4/3, S5/1
  T_carrier_us_AXI/1 -> T_carrier_us_rd_AXI/1, Counter Ctrl/3(T_carrier_us)
  Switch7/1 -> Switch3/1
  min_pulse_width_AXI/1 -> LimitPulseWidth/2(min_pulse_width), LimitPulseWidth2/2(min_pulse_width), LimitPulseWidth1/2(min_pulse_width), min_pulse_width_rd_AXI/1
  Counter Ctrl/3(Period_CenterMax) -> Index Vector/3, MinOrMax/1, Triangle_Max/1, Scope/4
  Counter Ctrl/4(Period_CenterMin) -> Scope/5, Triangle_Min/1, MinOrMax/2, Index Vector/2
  Index Vector/1 -> Switch/2, Switch1/2, Switch13/2, Switch2/2, Switch12/2, Switch11/2, applied_new_reference_value/1  "Allow (MIN,MAX or assymetrical) anew reference value"
  triangle_in/1 -> Delay4/1
  count_src_ext_AXI/1 -> Switch10/2
  HDL Counter2/1 -> Counter Ctrl/1(hdl_cnt)
  Delay4/1 -> Switch10/1
  triangle_shift_HB1_AXI/1 -> Switch11/1
  Triangle shift/1(triangle_sig) -> Scope5/3, Relational Operator/1, Scope1/2
  Triangle shift1/1(triangle_sig) -> Relational Operator1/1
  Switch10/1 -> Triangle shift1/1(triangle_in), Scope2/1, Switch6/2, Scope4/1, Triangle shift2/1(triangle_in), Scope1/1, Triangle shift/1(triangle_in)
  Triangle shift2/1(triangle_sig) -> Relational Operator2/1
  Switch11/1 -> Triangle shift/2(triangle_shift), Delay3/1
  Delay3/1 -> Switch11/3
  Switch12/1 -> Triangle shift1/2(triangle_shift), Delay5/1
  Delay5/1 -> Switch12/3
  triangle_shift_HB2_AXI/1 -> Switch12/1
  Switch13/1 -> Triangle shift2/2(triangle_shift), Delay6/1
  Delay6/1 -> Switch13/3
  triangle_shift_HB3_AXI/1 -> Switch13/1
  MinOrMax/1 -> Index Vector/4
  PWM_trigger_source_AXI/1 -> Index Vector/1
  counter_reset/1 -> HDL Counter2/1

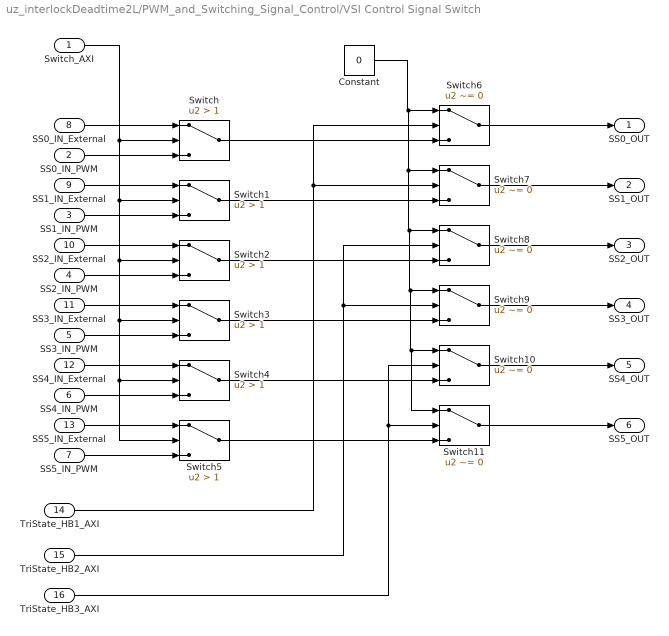
== system uz_interlockDeadtime2L/PWM_and_Switching_Signal_Control/VSI Control Signal Switch ==
  Switch_AXI : Inport
  SS0_IN_PWM : Inport  Port=2
  SS1_IN_PWM : Inport  Port=3
  SS2_IN_PWM : Inport  Port=4
  SS3_IN_PWM : Inport  Port=5
  SS4_IN_PWM : Inport  Port=6
  SS5_IN_PWM : Inport  Port=7
  SS0_IN_External : Inport  Port=8
  SS1_IN_External : Inport  Port=9
  SS2_IN_External : Inport  Port=10
  SS3_IN_External : Inport  Port=11
  SS4_IN_External : Inport  Port=12
  SS5_IN_External : Inport  Port=13
  TriState_HB1_AXI : Inport  Port=14
  TriState_HB2_AXI : Inport  Port=15
  TriState_HB3_AXI : Inport  Port=16
  Constant : Constant  Value=0  OutDataTypeStr=boolean  SampleTime=T_FPGA_clk
  Switch{,1..5} (6 alike) : Switch  Criteria=u2 > Threshold  Threshold=1  SaturateOnIntegerOverflow=off  InputSameDT=off
  Switch{6..11} (6 alike) : Switch  Criteria=u2 ~= 0  Threshold=1  SaturateOnIntegerOverflow=off  InputSameDT=off
  SS0_OUT : Outport  VectorParamsAs1DForOutWhenUnconnected=off
  SS1_OUT : Outport  Port=2  VectorParamsAs1DForOutWhenUnconnected=off
  SS2_OUT : Outport  Port=3  VectorParamsAs1DForOutWhenUnconnected=off
  SS3_OUT : Outport  Port=4  VectorParamsAs1DForOutWhenUnconnected=off
  SS4_OUT : Outport  Port=5  VectorParamsAs1DForOutWhenUnconnected=off
  SS5_OUT : Outport  Port=6  VectorParamsAs1DForOutWhenUnconnected=off
  wires:
  Switch_AXI/1 -> Switch4/2, Switch5/2, Switch3/2, Switch2/2, Switch1/2, Switch/2
  Switch5/1 -> Switch11/3
  Switch/1 -> Switch6/3
  Switch3/1 -> Switch9/3
  Switch2/1 -> Switch8/3
  Switch1/1 -> Switch7/3
  Switch4/1 -> Switch10/3
  SS0_IN_PWM/1 -> Switch/3
  SS0_IN_External/1 -> Switch/1
  SS1_IN_External/1 -> Switch1/1
  SS1_IN_PWM/1 -> Switch1/3
  SS2_IN_External/1 -> Switch2/1
  SS2_IN_PWM/1 -> Switch2/3
  SS3_IN_External/1 -> Switch3/1
  SS3_IN_PWM/1 -> Switch3/3
  SS4_IN_External/1 -> Switch4/1
  SS4_IN_PWM/1 -> Switch4/3
  SS5_IN_External/1 -> Switch5/1
  SS5_IN_PWM/1 -> Switch5/3
  TriState_HB3_AXI/1 -> Switch10/2, Switch11/2
  TriState_HB2_AXI/1 -> Switch8/2, Switch9/2
  TriState_HB1_AXI/1 -> Switch6/2, Switch7/2
  Switch11/1 -> SS5_OUT/1
  Switch10/1 -> SS4_OUT/1
  Switch9/1 -> SS3_OUT/1
  Switch8/1 -> SS2_OUT/1
  Switch7/1 -> SS1_OUT/1
  Switch6/1 -> SS0_OUT/1
  Constant/1 -> Switch11/1, Switch10/1, Switch9/1, Switch8/1, Switch7/1, Switch6/1

== system uz_interlockDeadtime2L/uz_interlockDeadtime2L/DeadtimeModule ==
  note: Resets the counter at a falling edge
  note: This delay is only used to improve timing (Pipeline) and is not related to the function of the module!
  In1 : Inport  Partition=on  PartitionDimension=1  PartitionWidth=1  PartitionOffset=0
  DelayCycles : Inport  Port=2
  Delay2 : Delay  DelayLength=1  ExternalReset=Level
      settings: InputPortMap=u0,r5
  Detect Fall Nonpositive2 : simulink/Logic and Bit Operations/Detect Fall Nonpositive  vinit=0  OutDataTypeStr=boolean
  For Each : ForEach  DisableCoverage=on
  HDL Counter : hdlsllib/Sources/HDL Counter  CountType=Free running  CountInit=0  CountStep=1  CountMax=25  CountFromType=Initial value  CountFrom=0  CountResetPort=on  CountLoadPort=off  CountEnbPort=on  CountDirPort=off  CountHitOutputPort=off  CountDataType=Unsigned  CountWordLen=10  CountFracLen=0  CountSampTime=-1
  Logical Operator10 : Logic  AllPortsSameDT=off  OutDataTypeStr=boolean
  PipelineDelay1 : Delay  DelayLength=1
  Relational Operator : RelationalOperator  Operator===  OutDataTypeStr=boolean  RndMeth=Simplest  InputSameDT=off
  Switch : Switch  Criteria=u2 ~= 0  Threshold=1  SaturateOnIntegerOverflow=off  InputSameDT=off
  gate_delay_out : Outport  ConcatenationDimension=1
  wires:
  In1/1 -> Logical Operator10/1, Switch/1, HDL Counter/2, Detect Fall Nonpositive2/1
  DelayCycles/1 -> Relational Operator/1
  Delay2/1 -> Switch/3
  HDL Counter/1 -> Relational Operator/2
  Detect Fall Nonpositive2/1 -> PipelineDelay1/1
  Relational Operator/1 -> Switch/2
  PipelineDelay1/1 -> HDL Counter/1, Delay2/2
  Switch/1 -> Delay2/1, Logical Operator10/2
  Logical Operator10/1 -> gate_delay_out/1

== system uz_interlockDeadtime2L/uz_interlockDeadtime2L/EnableOutputModule ==
  gate_delay_out : Inport  Partition=on  PartitionDimension=1  PartitionWidth=1  PartitionOffset=0
  enable : Inport  Port=2
  AND : Logic  AllPortsSameDT=off  OutDataTypeStr=boolean
  For Each : ForEach  DisableCoverage=on
  gate_enable_out : Outport  ConcatenationDimension=1
  wires:
  enable/1 -> AND/2
  gate_delay_out/1 -> AND/1
  AND/1 -> gate_enable_out/1

== system uz_interlockDeadtime2L/uz_interlockDeadtime2L/InterlockModule ==
  In1 : Inport  Partition=on  PartitionDimension=1  PartitionWidth=2  PartitionOffset=0
  Demux : Demux  Outputs=2
  For Each : ForEach  DisableCoverage=on
  Logical Operator1 : Logic  AllPortsSameDT=off  OutDataTypeStr=boolean
  Logical Operator2 : Logic  AllPortsSameDT=off  OutDataTypeStr=boolean
  Logical Operator3 : Logic  Operator=NOT  AllPortsSameDT=off  OutDataTypeStr=boolean
  Logical Operator4 : Logic  Operator=NOT  AllPortsSameDT=off  OutDataTypeStr=boolean
  Mux : Mux  Inputs=2
  gate_delay_out : Outport  ConcatenationDimension=1
  wires:
  Demux/1 -> Logical Operator4/1, Logical Operator2/1
  Logical Operator1/1 -> Mux/2  "interlock_bot_out"
  Demux/2 -> Logical Operator1/2, Logical Operator3/1
  Logical Operator3/1 -> Logical Operator2/2
  Logical Operator2/1 -> Mux/1  "PWM_AH"
  Logical Operator4/1 -> Logical Operator1/1
  Mux/1 -> gate_delay_out/1
  In1/1 -> Demux/1

== system uz_interlockDeadtime2L/uz_interlockDeadtime2L/InverseBotSwitchModule ==
  gate_delay_out : Inport  Partition=on  PartitionDimension=1  PartitionWidth=2  PartitionOffset=0
  inverse_bottom_switch : Inport  Port=2
  Demux : Demux  Outputs=2
  For Each : ForEach  DisableCoverage=on
  Index Vector : MultiPortSwitch  DataPortOrder=Zero-based contiguous  Inputs=2  zeroidx=on  SaturateOnIntegerOverflow=off  InputSameDT=off
  Mux : Mux  Inputs=2
  NOT : Logic  Operator=NOT  AllPortsSameDT=off  OutDataTypeStr=boolean
  PipeDelay : Delay  DelayLength=1
  gate_enable_out : Outport  ConcatenationDimension=1
  wires:
  PipeDelay/1 -> Index Vector/1
  Demux/2 -> Index Vector/2, NOT/1
  Index Vector/1 -> Mux/2
  inverse_bottom_switch/1 -> PipeDelay/1
  Demux/1 -> Mux/1
  NOT/1 -> Index Vector/3
  Mux/1 -> gate_enable_out/1
  gate_delay_out/1 -> Demux/1

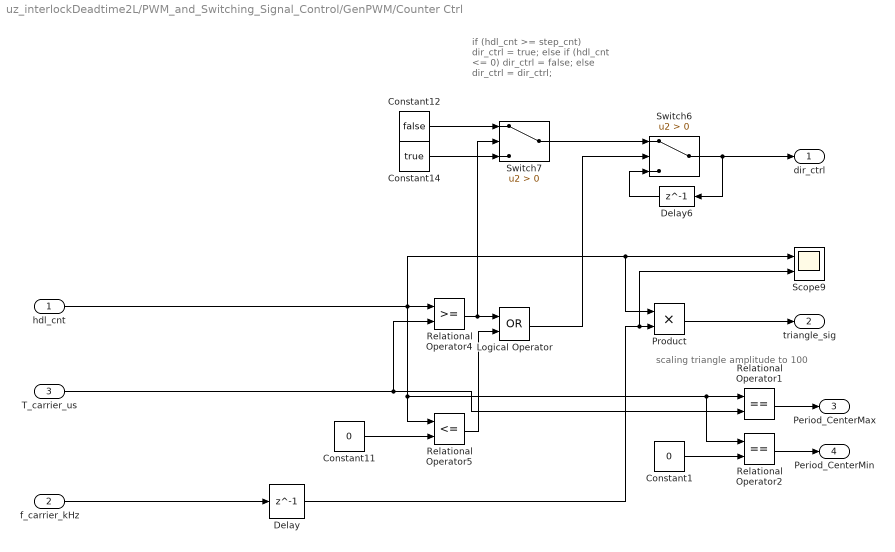
== system uz_interlockDeadtime2L/PWM_and_Switching_Signal_Control/GenPWM/Counter Ctrl ==
  note: if (hdl_cnt >= step_cnt)
      | 	dir_ctrl = true;
      | else if (hdl_cnt <= 0)
      | 	dir_ctrl = false;
      | else
      | 	dir_ctrl = dir_ctrl;
  note: scaling triangle amplitude to 100
  hdl_cnt : Inport
  f_carrier_kHz : Inport  Port=2
  T_carrier_us : Inport  Port=3
  Constant1 : Constant  Value=0  OutDataTypeStr=fixdt(0,20,0)  SampleTime=T_FPGA_clk
  Constant11 : Constant  Value=0  OutDataTypeStr=fixdt(0,20,0)  SampleTime=T_FPGA_clk
  Constant12 : Constant  Value=false  SampleTime=T_FPGA_clk
  Constant14 : Constant  Value=true  SampleTime=T_FPGA_clk
  Delay : Delay  DelayLength=1
  Delay6 : Delay  DelayLength=1
  Logical Operator : Logic  Operator=OR  AllPortsSameDT=off  OutDataTypeStr=boolean
  Product : Product  OutDataTypeStr=fixdt(0,18,17)
  Relational Operator1 : RelationalOperator  Operator===  OutDataTypeStr=boolean  InputSameDT=off
  Relational Operator2 : RelationalOperator  Operator===  OutDataTypeStr=boolean  InputSameDT=off
  Relational Operator4 : RelationalOperator  OutDataTypeStr=boolean  InputSameDT=off
  Relational Operator5 : RelationalOperator  Operator=<=  OutDataTypeStr=boolean  InputSameDT=off
  Scope9 : Scope  NumInputPorts=2
  Switch6 : Switch  Criteria=u2 > Threshold  SaturateOnIntegerOverflow=off  InputSameDT=off
  Switch7 : Switch  Criteria=u2 > Threshold  SaturateOnIntegerOverflow=off  InputSameDT=off
  dir_ctrl : Outport  VectorParamsAs1DForOutWhenUnconnected=off
  triangle_sig : Outport  Port=2  VectorParamsAs1DForOutWhenUnconnected=off
  Period_CenterMax : Outport  Port=3  VectorParamsAs1DForOutWhenUnconnected=off
  Period_CenterMin : Outport  Port=4  VectorParamsAs1DForOutWhenUnconnected=off
  wires:
  hdl_cnt/1 -> Relational Operator2/1, Relational Operator1/1, Relational Operator5/1, Relational Operator4/1, Product/1, Scope9/1
  Switch6/1 -> Delay6/1, dir_ctrl/1
  Relational Operator4/1 -> Switch7/2, Logical Operator/1
  Relational Operator5/1 -> Logical Operator/2
  Constant11/1 -> Relational Operator5/2
  Logical Operator/1 -> Switch6/2
  Switch7/1 -> Switch6/1
  Constant12/1 -> Switch7/1
  Constant14/1 -> Switch7/3
  Delay6/1 -> Switch6/3
  T_carrier_us/1 -> Relational Operator4/2, Relational Operator1/2
  f_carrier_kHz/1 -> Delay/1
  Delay/1 -> Scope9/2, Product/2
  Relational Operator1/1 -> Period_CenterMax/1
  Relational Operator2/1 -> Period_CenterMin/1
  Constant1/1 -> Relational Operator2/2
  Product/1 -> triangle_sig/1

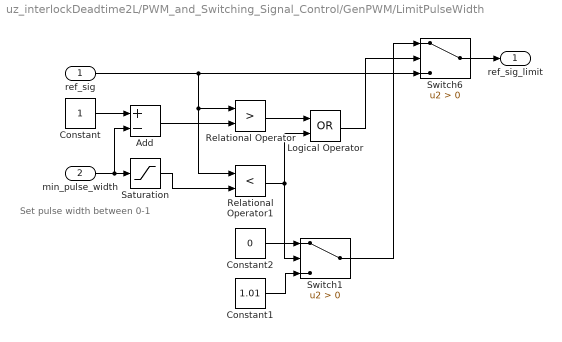
== system uz_interlockDeadtime2L/PWM_and_Switching_Signal_Control/GenPWM/LimitPulseWidth ==
  note: Set pulse width between 0-1
  ref_sig : Inport
  min_pulse_width : Inport  Port=2
  Add : Sum  Inputs=+-  OutDataTypeStr=Inherit: Same as first input
  Constant : Constant  OutDataTypeStr=fixdt(1,18,16)  SampleTime=T_FPGA_clk
  Constant1 : Constant  Value=1.01  OutDataTypeStr=fixdt(1,18,16)  SampleTime=T_FPGA_clk
  Constant2 : Constant  Value=0  OutDataTypeStr=fixdt(1,18,16)  SampleTime=T_FPGA_clk
  Logical Operator : Logic  Operator=OR  AllPortsSameDT=off  OutDataTypeStr=boolean
  Relational Operator : RelationalOperator  Operator=>  OutDataTypeStr=boolean  InputSameDT=off
  Relational Operator1 : RelationalOperator  Operator=<  OutDataTypeStr=boolean  InputSameDT=off
  Saturation : Saturate  UpperLimit=1  LowerLimit=0  OutDataTypeStr=fixdt(1,18,16)
  Switch1 : Switch  Criteria=u2 > Threshold  SaturateOnIntegerOverflow=off  InputSameDT=off
  Switch6 : Switch  Criteria=u2 > Threshold  SaturateOnIntegerOverflow=off  InputSameDT=off
  ref_sig_limit : Outport  VectorParamsAs1DForOutWhenUnconnected=off
  wires:
  Constant/1 -> Add/1
  min_pulse_width/1 -> Add/2, Saturation/1
  Add/1 -> Relational Operator/2
  ref_sig/1 -> Switch6/3, Relational Operator/1, Relational Operator1/1
  Relational Operator/1 -> Logical Operator/1
  Relational Operator1/1 -> Logical Operator/2, Switch1/2
  Logical Operator/1 -> Switch6/2
  Constant1/1 -> Switch1/3
  Switch1/1 -> Switch6/1
  Constant2/1 -> Switch1/1
  Switch6/1 -> ref_sig_limit/1
  Saturation/1 -> Relational Operator1/2

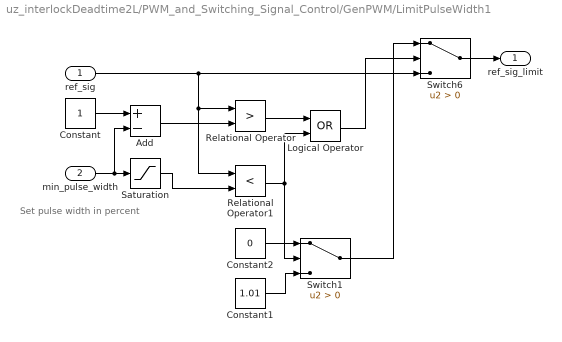
== system uz_interlockDeadtime2L/PWM_and_Switching_Signal_Control/GenPWM/LimitPulseWidth1 ==
  note: Set pulse width in percent
  ref_sig : Inport
  min_pulse_width : Inport  Port=2
  Add : Sum  Inputs=+-  OutDataTypeStr=Inherit: Same as first input
  Constant : Constant  OutDataTypeStr=fixdt(1,18,16)  SampleTime=T_FPGA_clk
  Constant1 : Constant  Value=1.01  OutDataTypeStr=fixdt(1,18,16)  SampleTime=T_FPGA_clk
  Constant2 : Constant  Value=0  OutDataTypeStr=fixdt(1,18,16)  SampleTime=T_FPGA_clk
  Logical Operator : Logic  Operator=OR  AllPortsSameDT=off  OutDataTypeStr=boolean
  Relational Operator : RelationalOperator  Operator=>  OutDataTypeStr=boolean  InputSameDT=off
  Relational Operator1 : RelationalOperator  Operator=<  OutDataTypeStr=boolean  InputSameDT=off
  Saturation : Saturate  UpperLimit=1  LowerLimit=0  OutDataTypeStr=fixdt(1,18,16)
  Switch1 : Switch  Criteria=u2 > Threshold  SaturateOnIntegerOverflow=off  InputSameDT=off
  Switch6 : Switch  Criteria=u2 > Threshold  SaturateOnIntegerOverflow=off  InputSameDT=off
  ref_sig_limit : Outport  VectorParamsAs1DForOutWhenUnconnected=off
  wires:
  Constant/1 -> Add/1
  min_pulse_width/1 -> Add/2, Saturation/1
  Add/1 -> Relational Operator/2
  ref_sig/1 -> Switch6/3, Relational Operator/1, Relational Operator1/1
  Relational Operator/1 -> Logical Operator/1
  Relational Operator1/1 -> Logical Operator/2, Switch1/2
  Logical Operator/1 -> Switch6/2
  Constant1/1 -> Switch1/3
  Switch1/1 -> Switch6/1
  Constant2/1 -> Switch1/1
  Switch6/1 -> ref_sig_limit/1
  Saturation/1 -> Relational Operator1/2

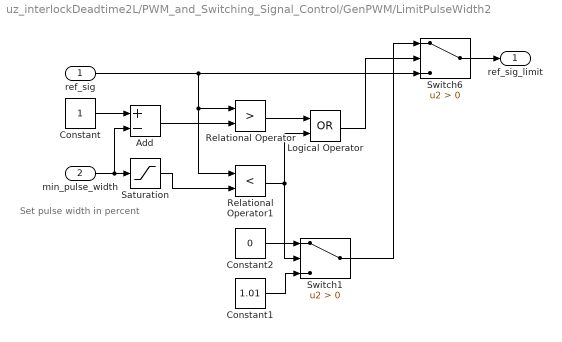
== system uz_interlockDeadtime2L/PWM_and_Switching_Signal_Control/GenPWM/LimitPulseWidth2 ==
  note: Set pulse width in percent
  ref_sig : Inport
  min_pulse_width : Inport  Port=2
  Add : Sum  Inputs=+-  OutDataTypeStr=Inherit: Same as first input
  Constant : Constant  OutDataTypeStr=fixdt(1,18,16)  SampleTime=T_FPGA_clk
  Constant1 : Constant  Value=1.01  OutDataTypeStr=fixdt(1,18,16)  SampleTime=T_FPGA_clk
  Constant2 : Constant  Value=0  OutDataTypeStr=fixdt(1,18,16)  SampleTime=T_FPGA_clk
  Logical Operator : Logic  Operator=OR  AllPortsSameDT=off  OutDataTypeStr=boolean
  Relational Operator : RelationalOperator  Operator=>  OutDataTypeStr=boolean  InputSameDT=off
  Relational Operator1 : RelationalOperator  Operator=<  OutDataTypeStr=boolean  InputSameDT=off
  Saturation : Saturate  UpperLimit=1  LowerLimit=0  OutDataTypeStr=fixdt(1,18,16)
  Switch1 : Switch  Criteria=u2 > Threshold  SaturateOnIntegerOverflow=off  InputSameDT=off
  Switch6 : Switch  Criteria=u2 > Threshold  SaturateOnIntegerOverflow=off  InputSameDT=off
  ref_sig_limit : Outport  VectorParamsAs1DForOutWhenUnconnected=off
  wires:
  Constant/1 -> Add/1
  min_pulse_width/1 -> Add/2, Saturation/1
  Add/1 -> Relational Operator/2
  ref_sig/1 -> Switch6/3, Relational Operator/1, Relational Operator1/1
  Relational Operator/1 -> Logical Operator/1
  Relational Operator1/1 -> Logical Operator/2, Switch1/2
  Logical Operator/1 -> Switch6/2
  Constant1/1 -> Switch1/3
  Switch1/1 -> Switch6/1
  Constant2/1 -> Switch1/1
  Switch6/1 -> ref_sig_limit/1
  Saturation/1 -> Relational Operator1/2

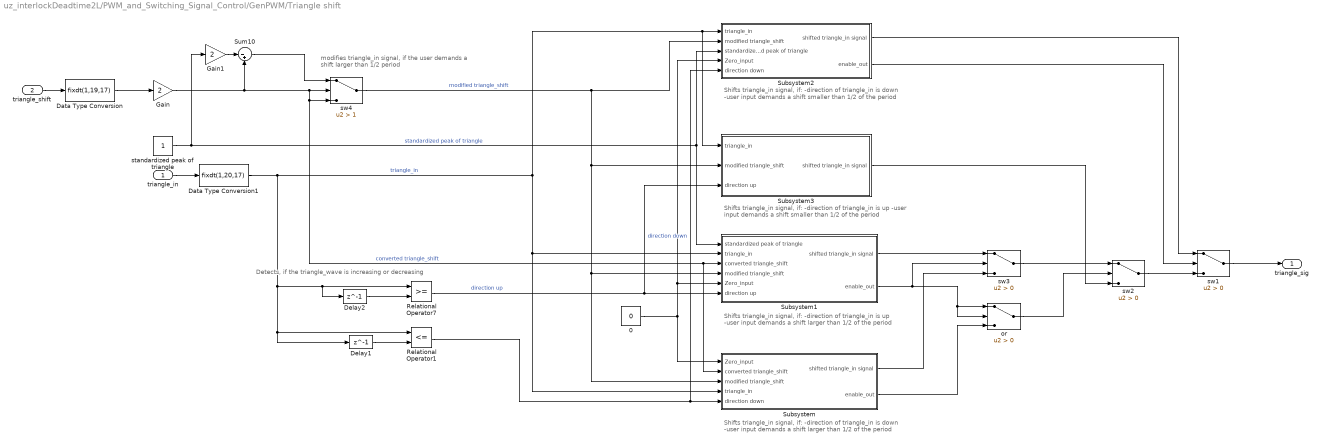
== system uz_interlockDeadtime2L/PWM_and_Switching_Signal_Control/GenPWM/Triangle shift ==
  note: modifies triangle_in signal,
      | if the user demands a shift larger than 1/2 period
  note: Detects, if the triangle_wave is increasing or decreasing
  note: Shifts triangle_in signal, if:
      | -direction of triangle_in is down
      | -user input demands a shift larger than 1/2 of the period
  note: Shifts triangle_in signal, if:
      | -direction of triangle_in is up
      | -user input demands a shift larger than 1/2 of the period
  note: Shifts triangle_in signal, if:
      | -direction of triangle_in is up
      | -user input demands a shift smaller than 1/2 of the period
  note: Shifts triangle_in signal, if:
      | -direction of triangle_in is down
      | -user input demands a shift smaller than 1/2 of the period
  triangle_in : Inport
  triangle_shift : Inport  Port=2
  0 : Constant  Value=0  OutDataTypeStr=boolean  SampleTime=T_FPGA_clk
  Data Type Conversion : DataTypeConversion  OutDataTypeStr=fixdt(1,19,17)  SaturateOnIntegerOverflow=off  RndMeth=Floor
  Data Type Conversion1 : DataTypeConversion  OutDataTypeStr=fixdt(1,20,17)  SaturateOnIntegerOverflow=off  RndMeth=Floor
  Delay1 : Delay  DelayLength=1
  Delay2 : Delay  DelayLength=1
  Gain : Gain  Gain=2  OutDataTypeStr=fixdt(1,20,17)
  Gain1 : Gain  Gain=2  OutDataTypeStr=fixdt(1,20,17)
  Relational Operator1 : RelationalOperator  Operator=<=  OutDataTypeStr=boolean  InputSameDT=off
  Relational Operator7 : RelationalOperator  OutDataTypeStr=boolean  InputSameDT=off
  Subsystem : Subsystem
  Subsystem1 : Subsystem
  Subsystem2 : Subsystem
  Subsystem3 : Subsystem
  Sum10 : Sum  Inputs=|-+  OutDataTypeStr=fixdt(1,20,17)
  or : Switch  Criteria=u2 > Threshold  SaturateOnIntegerOverflow=off  InputSameDT=off
  standardized peak of triangle : Constant  OutDataTypeStr=fixdt(0,21,17)  SampleTime=T_FPGA_clk
  sw1 : Switch  Criteria=u2 > Threshold  OutDataTypeStr=fixdt(1,18,16)  SaturateOnIntegerOverflow=off  InputSameDT=off
  sw2 : Switch  Criteria=u2 > Threshold  SaturateOnIntegerOverflow=off  InputSameDT=off
  sw3 : Switch  Criteria=u2 > Threshold  SaturateOnIntegerOverflow=off  InputSameDT=off
  sw4 : Switch  Criteria=u2 > Threshold  Threshold=1  OutDataTypeStr=fixdt(1,20,17)  SaturateOnIntegerOverflow=off  InputSameDT=off
  triangle_sig : Outport  VectorParamsAs1DForOutWhenUnconnected=off
  wires:
  Delay2/1 -> Relational Operator7/2
  Data Type Conversion1/1 -> Subsystem3/1(triangle_in), Subsystem2/1(triangle_in), Subsystem/4(triangle_in), Subsystem1/2(triangle_in), Relational Operator1/1, Delay1/1, Delay2/1, Relational Operator7/1  "triangle_in"
  sw3/1 -> sw2/1
  Relational Operator7/1 -> Subsystem1/6(direction up), Subsystem3/3(direction up)  "direction up"
  or/1 -> sw2/2
  sw4/1 -> Subsystem3/2(modified triangle_shift), Subsystem/3(modified triangle_shift), Subsystem1/4(modified triangle_shift), Subsystem2/2(modified triangle_shift)  "modified triangle_shift"
  Gain/1 -> Sum10/2, Subsystem/2(converted triangle_shift), Subsystem1/3(converted triangle_shift), sw4/3, sw4/2  "converted triangle_shift"
  Sum10/1 -> sw4/1
  sw1/1 -> triangle_sig/1
  standardized peak of triangle/1 -> Subsystem2/3(standardized peak of triangle), Subsystem1/1(standardized peak of triangle), Gain1/1  "standardized peak of triangle"
  triangle_shift/1 -> Data Type Conversion/1
  Gain1/1 -> Sum10/1
  sw2/1 -> sw1/3
  Data Type Conversion/1 -> Gain/1
  triangle_in/1 -> Data Type Conversion1/1
  Relational Operator1/1 -> Subsystem/5(direction down), Subsystem2/5(direction down)  "direction down"
  Delay1/1 -> Relational Operator1/2
  0/1 -> Subsystem2/4(Zero_input), Subsystem1/5(Zero_input), Subsystem/1(Zero_input)
  Subsystem/1(shifted triangle_in signal) -> sw3/3
  Subsystem/2(enable_out) -> or/3
  Subsystem1/2(enable_out) -> or/2, or/1, sw3/2
  Subsystem1/1(shifted triangle_in signal) -> sw3/1
  Subsystem2/1(shifted triangle_in signal) -> sw1/1
  Subsystem2/2(enable_out) -> sw1/2
  Subsystem3/1(shifted triangle_in signal) -> sw2/3
